simulink model "new_logic_trial"  (R2025a)
settings: Solver=VariableStepAuto  StartTime=0.0  StopTime=50  RelTol=1e-3
undefined symbols (not defined in the file): a
settings Model: Creator=Deepak  LastModifiedBy=Deepak

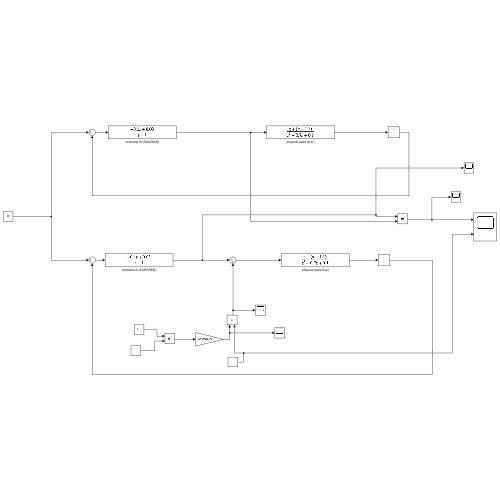
[thumbnail: Simulink's stored preview of the top-level diagram]
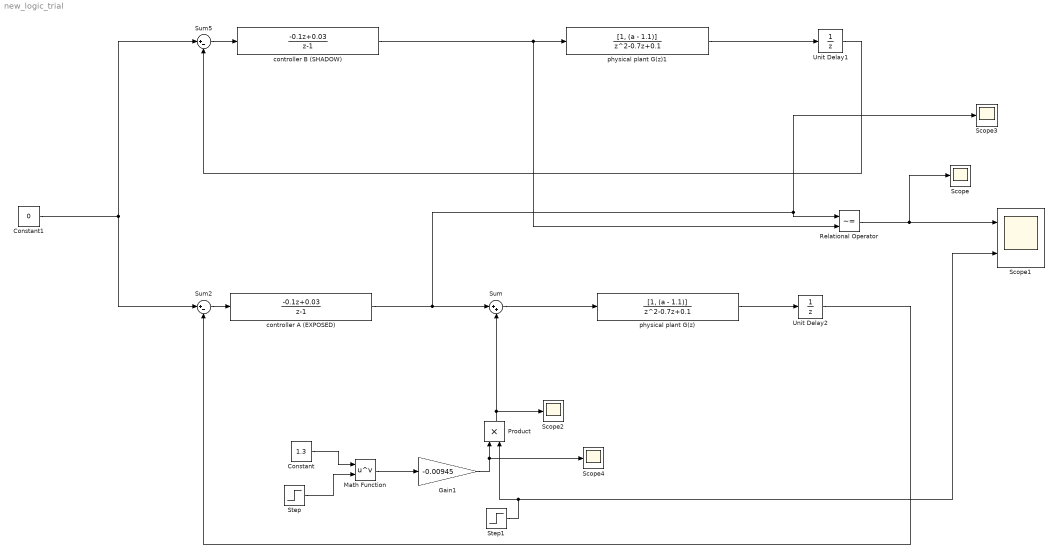
== system new_logic_trial ==
  Constant : Constant  Value=1.3
  Constant1 : Constant  Value=0
  Gain1 : Gain  Gain=-0.00945
  Math Function : Math  Operator=pow
  Product : Product
  Relational Operator : RelationalOperator  Operator=~=  OutDataTypeStr=boolean  RndMeth=Simplest  InputSameDT=off
  Scope{,2..4} (4 alike) : Scope
      Scope settings: ActiveDisplayYMinimum=-1  ActiveDisplayYMaximum=1
      Scope2 settings: ActiveDisplayYMinimum=-0.013820625000000001  ActiveDisplayYMaximum=0.0015356249999999997  DataLoggingVariableName=ScopeData2
      Scope3 settings: ActiveDisplayYMinimum=-0.015052293516499997  ActiveDisplayYMaximum=0.1127835881685  DataLoggingVariableName=ScopeData3
      Scope4 settings: ActiveDisplayYMinimum=-0.0012639375  ActiveDisplayYMaximum=-0.00090956250000000011  DataLoggingVariableName=ScopeData4
  Scope1 : Scope  NumInputPorts=2
      settings: ActiveDisplayYMinimum=-0.12499999999999997  ActiveDisplayYMaximum=1.125
  Step : Step  Time=20  SampleTime=1  VectorParams1D=off  ZeroCross=off
  Step1 : Step  Time=20  SampleTime=1  VectorParams1D=off  ZeroCross=off
  Sum : Sum  Inputs=|++
  Sum2 : Sum  Inputs=|+-
  Sum5 : Sum  Inputs=|+-
  Unit Delay1 : UnitDelay  InitialCondition=1  SampleTime=0.001  HasFrameUpgradeWarning=on
  Unit Delay2 : UnitDelay  InitialCondition=1  SampleTime=0.001  HasFrameUpgradeWarning=on
  controller A (EXPOSED) : DiscreteTransferFcn  Numerator=[-0.1, 0.03]  Denominator=[1, -1]
  controller B (SHADOW) : DiscreteTransferFcn  Numerator=[-0.1, 0.03]  Denominator=[1, -1]
  physical plant G(z) : DiscreteTransferFcn  Numerator=[1, (a - 1.1)]  Denominator=[1, -0.7, 0.1]
  physical plant G(z)1 : DiscreteTransferFcn  Numerator=[1, (a - 1.1)]  Denominator=[1, -0.7, 0.1]
  wires:
  Sum/1 -> physical plant G(z)/1
  Product/1 -> Sum/2, Scope2/1
  physical plant G(z)1/1 -> Unit Delay1/1
  Unit Delay2/1 -> Sum2/2
  controller A (EXPOSED)/1 -> Relational Operator/1, Scope3/1, Sum/1
  Sum2/1 -> controller A (EXPOSED)/1
  Step1/1 -> Scope1/2, Product/2
  Unit Delay1/1 -> Sum5/2
  Sum5/1 -> controller B (SHADOW)/1
  physical plant G(z)/1 -> Unit Delay2/1
  Step/1 -> Math Function/2
  Constant/1 -> Math Function/1
  Gain1/1 -> Product/1, Scope4/1
  controller B (SHADOW)/1 -> Relational Operator/2, physical plant G(z)1/1
  Constant1/1 -> Sum5/1, Sum2/1
  Math Function/1 -> Gain1/1
  Relational Operator/1 -> Scope/1, Scope1/1
